simulink model "Model"  (R2015a)
settings: Solver=ode1  StartTime=0.0  StopTime=Inf  FixedStep=0.001  RelTol=1e-3
PostLoadFcn:
  | , if any(exist('dsrtsu_mdlpostloadfcn', 'file') == [2, 3, 6]), try dsrtsu_mdlpostloadfcn('Execute', bdroot); catch fprintf('Error in PostLoadFcn (dsrtsu_mdlpostloadfcn) for model "%s":\n %s\n', bdroot, lasterr); end, end,
libraries: rtilib1104 x9, simulink x6, simulink_extras x3
settings Model: DSRTSU_INTERNAL_RTI_VER=460  DSRTSU_INTERNAL_RTI_TYPE=rti1104  DSRTSU_INTERNAL_RTIFPGA=50  Creator=k19p800a  LastModifiedBy=k19p800a
settings OptimizationCC: BlockReduction=off  OptimizeBlockIOStorage=off  BufferReuse=off  GlobalBufferReuse=off  ExpressionFolding=off  LocalBlockOutputs=off
settings HardwareCC: ProdIntDivRoundTo=Zero  ProdEndianess=BigEndian  ProdHWDeviceType=Generic->Custom  TargetIntDivRoundTo=Zero  TargetEndianess=BigEndian  TargetHWDeviceType=Generic->Custom
settings RTWCC: SystemTargetFile=rti1104.tlc  MakeCommand=make_rti  TemplateMakefile=rti1104.tmf  Description=dSPACE DS1104 Hardware Platform
settings STFCustomTargetCC: GenerateSampleERTMain=off  ParMdlRefBuildCompliant=on  GeneratePreprocessorConditionals=Disable all  ERTCustomFileBanners=off  SupportNonInlinedSFcns=on  SupportVariableSizeSignals=off  MATLABClassNameForMDSCustomization=Simulink.SoftwareTarget.GRTCustomization  GRTInterface=on  SystemTargetFile=rti1104.tlc
settings GRTTargetCC: CompOptLevelCompliant=off  ConcurrentExecutionCompliant=off  CombineOutputUpdateFcns=off  MatFileLogging=off  CPPClassGenCompliant=off  GRTInterface=on  ExtModeMexFile=noextcomm

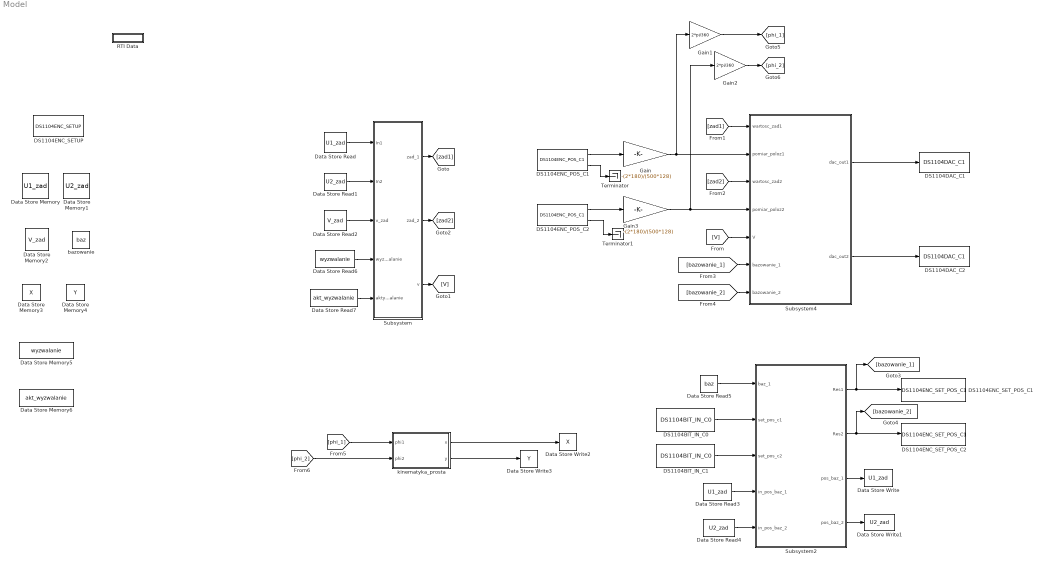
== system Model ==
  DS1104BIT_IN_C0 : rtilib1104/DS1104 MASTER PPC/DS1104BIT_IN_C0  ChannelNo=0  Reserved1=[]  Reserved2=[]  Reserved3=[]  Reserved4=[]  DialogFcn=gui1104bit_in  UnitName={'DS1104BIT_IN_C'}  UnitValues={ 0 }  DSProperties=struct('RTI',struct('Version',uint32(1),'BlockType',struct('isSLSource',uint8(1),'isSLSink',uint8(0),'isHWSource',uint8(1),'isHWSink',uint8(0),'isSetup',uint8(0),'isInline',uint8(1),'isNonInline',uint8(0),'isInterrupt',uint8(0),'isChannelwise',uint8(1)),'IOBoardType','DS1104MASTER','UnitType','BIT','Identifier','BITINCH','DialogType','ML','BlockSet','NONE','SlaveProcessor','NONE'))
  DS1104BIT_IN_C1 : rtilib1104/DS1104 MASTER PPC/DS1104BIT_IN_C0  ChannelNo=1  Reserved1=[]  Reserved2=[]  Reserved3=[]  Reserved4=[]  DialogFcn=gui1104bit_in  UnitName={'DS1104BIT_IN_C'}  UnitValues={ 1 }  DSProperties=struct('RTI',struct('Version',uint32(1),'BlockType',struct('isSLSource',uint8(1),'isSLSink',uint8(0),'isHWSource',uint8(1),'isHWSink',uint8(0),'isSetup',uint8(0),'isInline',uint8(1),'isNonInline',uint8(0),'isInterrupt',uint8(0),'isChannelwise',uint8(1)),'IOBoardType','DS1104MASTER','UnitType','BIT','Identifier','BITINCH','DialogType','ML','BlockSet','NONE','SlaveProcessor','NONE'))
  DS1104DAC_C1 : rtilib1104/DS1104 MASTER PPC/DS1104DAC_C1  ChannelNo=1  InitValue=0  TermMode=0  TermValue=0  Reserved1=[]  Reserved2=[]  Reserved3=[]  Reserved4=[]  DialogFcn=gui1104dac  UnitName={ 'DS1104DAC_C'}  UnitValues={ 1 }  DSProperties=struct('RTI',struct('Version',uint32(1),'BlockType',struct('isSLSource',uint8(0),'isSLSink',uint8(1),'isHWSource',uint8(0),'isHWSink',uint8(1),'isSetup',uint8(0),'isInline',uint8(1),'isNonInline',uint8(0),'isInterrupt',uint8(0),'isChannelwise',uint8(1)),'IOBoardType','DS1104MASTER','UnitType','DAC','Identifier','DAC','DialogType','ML','BlockSet','NONE','SlaveProcessor','NONE'))
  DS1104DAC_C2 : rtilib1104/DS1104 MASTER PPC/DS1104DAC_C1  ChannelNo=2  InitValue=0  TermMode=0  TermValue=0  Reserved1=[]  Reserved2=[]  Reserved3=[]  Reserved4=[]  DialogFcn=gui1104dac  UnitName={ 'DS1104DAC_C'}  UnitValues={2}  DSProperties=struct('RTI',struct('Version',uint32(1),'BlockType',struct('isSLSource',uint8(0),'isSLSink',uint8(1),'isHWSource',uint8(0),'isHWSink',uint8(1),'isSetup',uint8(0),'isInline',uint8(1),'isNonInline',uint8(0),'isInterrupt',uint8(0),'isChannelwise',uint8(1)),'IOBoardType','DS1104MASTER','UnitType','DAC','Identifier','DAC','DialogType','ML','BlockSet','NONE','SlaveProcessor','NONE'))
  DS1104ENC_POS_C1 : rtilib1104/DS1104 MASTER PPC/DS1104ENC_POS_C1  ChannelNo=1  PosValue=0  Reserved1=[]  Reserved2=[]  Reserved3=[]  Reserved4=[]  DialogFcn=gui1104enc_pos  UnitName={'DS1104ENC_POS_C'}  UnitValues={ 1 }  DSProperties=struct('RTI',struct('Version',uint32(1),'BlockType',struct('isSLSource',uint8(1),'isSLSink',uint8(0),'isHWSource',uint8(1),'isHWSink',uint8(0),'isSetup',uint8(0),'isInline',uint8(1),'isNonInline',uint8(0),'isInterrupt',uint8(0),'isChannelwise',uint8(1)),'IOBoardType','DS1104MASTER','UnitType','ENC','Identifier','ENCPOSCH','DialogType','ML','BlockSet','NONE','SlaveProcessor','NONE'))
  DS1104ENC_POS_C2 : rtilib1104/DS1104 MASTER PPC/DS1104ENC_POS_C1  ChannelNo=2  PosValue=0  Reserved1=[]  Reserved2=[]  Reserved3=[]  Reserved4=[]  DialogFcn=gui1104enc_pos  UnitName={'DS1104ENC_POS_C'}  UnitValues={2}  DSProperties=struct('RTI',struct('Version',uint32(1),'BlockType',struct('isSLSource',uint8(1),'isSLSink',uint8(0),'isHWSource',uint8(1),'isHWSink',uint8(0),'isSetup',uint8(0),'isInline',uint8(1),'isNonInline',uint8(0),'isInterrupt',uint8(0),'isChannelwise',uint8(1)),'IOBoardType','DS1104MASTER','UnitType','ENC','Identifier','ENCPOSCH','DialogType','ML','BlockSet','NONE','SlaveProcessor','NONE'))
  DS1104ENC_SETUP : rtilib1104/DS1104 MASTER PPC/DS1104ENC_SETUP  Reserved1=[]  Reserved2=[]  Reserved3=[]  Reserved4=[]  DialogFcn=gui1104enc_setup  UnitName={'DS1104ENC_SETUP'}  UnitValues={ [] }  DSProperties=struct('RTI',struct('Version',uint32(1),'BlockType',struct('isSLSource',uint8(0),'isSLSink',uint8(0),'isHWSource',uint8(0),'isHWSink',uint8(0),'isSetup',uint8(0),'isInline',uint8(1),'isNonInline',uint8(0),'isInterrupt',uint8(0),'isChannelwise',uint8(0)),'IOBoardType','DS1104MASTER','UnitType','ENC','Identifier','ENCSETUP','DialogType','ML','BlockSet','NONE','SlaveProcessor','NONE'))
      settings: SignalType=[0 0]
  DS1104ENC_SET_POS_C1 : rtilib1104/DS1104 MASTER PPC/DS1104ENC_SET_POS_C1  ChannelNo=1  PosValue=0  Reserved1=[]  Reserved2=[]  Reserved3=[]  Reserved4=[]  DialogFcn=gui1104enc_set_pos  UnitName={'DS1104ENC_SET_POS_C'}  UnitValues={ 1 }  DSProperties=struct('RTI',struct('Version',uint32(1),'BlockType',struct('isSLSource',uint8(0),'isSLSink',uint8(1),'isHWSource',uint8(0),'isHWSink',uint8(1),'isSetup',uint8(0),'isInline',uint8(1),'isNonInline',uint8(0),'isInterrupt',uint8(0),'isChannelwise',uint8(1)),'IOBoardType','DS1104MASTER','UnitType','ENC','Identifier','ENCRESET','DialogType','ML','BlockSet','NONE','SlaveProcessor','NONE'))
  DS1104ENC_SET_POS_C2 : rtilib1104/DS1104 MASTER PPC/DS1104ENC_SET_POS_C1  ChannelNo=2  PosValue=0  Reserved1=[]  Reserved2=[]  Reserved3=[]  Reserved4=[]  DialogFcn=gui1104enc_set_pos  UnitName={'DS1104ENC_SET_POS_C'}  UnitValues={2}  DSProperties=struct('RTI',struct('Version',uint32(1),'BlockType',struct('isSLSource',uint8(0),'isSLSink',uint8(1),'isHWSource',uint8(0),'isHWSink',uint8(1),'isSetup',uint8(0),'isInline',uint8(1),'isNonInline',uint8(0),'isInterrupt',uint8(0),'isChannelwise',uint8(1)),'IOBoardType','DS1104MASTER','UnitType','ENC','Identifier','ENCRESET','DialogType','ML','BlockSet','NONE','SlaveProcessor','NONE'))
  Data Store Memory : DataStoreMemory  DataStoreName=U1_zad  ReadBeforeWriteMsg=warning  WriteAfterWriteMsg=warning  WriteAfterReadMsg=warning
  Data Store Memory1 : DataStoreMemory  DataStoreName=U2_zad  ReadBeforeWriteMsg=warning  WriteAfterWriteMsg=warning  WriteAfterReadMsg=warning
  Data Store Memory2 : DataStoreMemory  DataStoreName=V_zad  ReadBeforeWriteMsg=warning  WriteAfterWriteMsg=warning  WriteAfterReadMsg=warning  InitialValue=25
  Data Store Memory3 : DataStoreMemory  DataStoreName=X  ReadBeforeWriteMsg=warning  WriteAfterWriteMsg=warning  WriteAfterReadMsg=warning
  Data Store Memory4 : DataStoreMemory  DataStoreName=Y  ReadBeforeWriteMsg=warning  WriteAfterWriteMsg=warning  WriteAfterReadMsg=warning
  Data Store Memory5 : DataStoreMemory  DataStoreName=wyzwalanie  ReadBeforeWriteMsg=warning  WriteAfterWriteMsg=warning  WriteAfterReadMsg=warning
  Data Store Memory6 : DataStoreMemory  DataStoreName=akt_wyzwalanie  ReadBeforeWriteMsg=warning  WriteAfterWriteMsg=warning  WriteAfterReadMsg=warning
  Data Store Read : DataStoreRead  DataStoreName=U1_zad
  Data Store Read1 : DataStoreRead  DataStoreName=U2_zad
  Data Store Read2 : DataStoreRead  DataStoreName=V_zad
  Data Store Read3 : DataStoreRead  DataStoreName=U1_zad
  Data Store Read4 : DataStoreRead  DataStoreName=U2_zad
  Data Store Read5 : DataStoreRead  DataStoreName=baz
  Data Store Read6 : DataStoreRead  DataStoreName=wyzwalanie
  Data Store Read7 : DataStoreRead  DataStoreName=akt_wyzwalanie
  Data Store Write : DataStoreWrite  DataStoreName=U1_zad
  Data Store Write1 : DataStoreWrite  DataStoreName=U2_zad
  Data Store Write2 : DataStoreWrite  DataStoreName=X
  Data Store Write3 : DataStoreWrite  DataStoreName=Y
  Gain : Gain  Gain=-(2*180)/(500*128)
  Gain1 : Gain  Gain=2*pi/360
  Gain2 : Gain  Gain=2*pi/360
  Gain3 : Gain  Gain=-(2*180)/(500*128)
  RTI Data : Subsystem  Tag=struct('RTIDataServer',struct('RTIDataServerVs','2','RTIModelDescription','struct(''main'',''Model'',''sub'','''',''isMp'',0)'))  LoadFcn="if exist('rtidc'), try,  rtidc('DataHostBlockClbLoad', gcbh); catch, disp(['Warning: ''LoadFcn'' for RTI Data block failed: ' lasterr]); end, end,"  mask(RTI_DATA_HOST){}
      mask help:
      | RTI Data Block.
      | This block is used by RTI to store internal model-dependent data.
      | Please keep this block on the root level of the model. Deleting this block will result in data loss.
      |
      | NEVER DELETE OR COPY THIS BLOCK!
      settings: CopyFcn="if exist('rtidc'), try,  rtidc('DataHostBlockClbCopy', gcbh); catch, disp(['Warning: ''CopyFcn'' for RTI Data block failed: ' lasterr]); end, end,"  DeleteFcn="if exist('rtidc'), try,  rtidc('DataHostBlockClbDelete', gcbh); catch, disp(['Warning: ''DeleteFcn'' for RTI Data block failed: ' lasterr]); end, end,"  ModelCloseFcn="if exist('rtidc'), try,  rtidc('DataHostBlockClbModelClose', gcbh); catch, disp(['Warning: ''ModelCloseFcn'' for RTI Data block failed: ' lasterr]); end, end,"  PreSaveFcn="if exist('rtidc'), try,  rtidc('DataHostBlockClbPreSave', gcbh); catch, disp(['Warning: ''PreSaveFcn'' for RTI Data block failed: ' lasterr]); end, end,"  PostSaveFcn="if exist('rtidc'), try,  rtidc('DataHostBlockClbPostSave', gcbh); catch, disp(['Warning: ''PostSaveFcn'' for RTI Data block failed: ' lasterr]); end, end,"  NameChangeFcn="if exist('rtidc'), try,  rtidc('DataHostBlockClbNameChange', gcbh); catch, disp(['Warning: ''NameChangeFcn'' for RTI Data block failed: ' lasterr]); end, end,"
      mask Help:
      | RTI Data Block.
      | This block is used by RTI to store internal model-dependent data.
      | Please keep this block on the root level of the model. Deleting this block will result in data loss.
      | 
      | NEVER DELETE OR COPY THIS BLOCK!
      mask Display:
      | text(0.5, 0.5, 'RTI Data', 'HorizontalAlignment', 'center');
      | plot([1 0]);
  Subsystem : Subsystem
  Subsystem2 : Subsystem
  Subsystem4 : Subsystem
  Terminator : Terminator
  Terminator1 : Terminator
  bazowanie : DataStoreMemory  DataStoreName=baz  ReadBeforeWriteMsg=warning  WriteAfterWriteMsg=warning  WriteAfterReadMsg=warning
  kinematyka_prosta : Subsystem
  wires:
  DS1104ENC_POS_C1/2 -> Terminator/1
  DS1104ENC_POS_C1/1 -> Gain/1
  Data Store Read/1 -> Subsystem/1(In1)
  Data Store Read1/1 -> Subsystem/2(In2)
  Data Store Read2/1 -> Subsystem/3(v_zad)
  Subsystem/1(zad_1) -> [zad1]
  DS1104ENC_POS_C2/1 -> Gain3/1
  DS1104ENC_POS_C2/2 -> Terminator1/1
  Gain/1 -> Gain1/1, Subsystem4/2(pomiar_poloz1)
  Gain3/1 -> Gain2/1, Subsystem4/4(pomiar_poloz2)
  Subsystem/3(v) -> [V]
  [V] -> Subsystem4/5(V)
  [zad1] -> Subsystem4/1(wartosc_zad1)
  Subsystem/2(zad_2) -> [zad2]
  [zad2] -> Subsystem4/3(wartosc_zad2)
  Subsystem2/3(pos_baz_1) -> Data Store Write/1
  Subsystem2/4(pos_baz_2) -> Data Store Write1/1
  Data Store Read3/1 -> Subsystem2/4(in_pos_baz_1)
  Data Store Read4/1 -> Subsystem2/5(in_pos_baz_2)
  Data Store Read5/1 -> Subsystem2/1(baz_1)
  Subsystem2/1(Res1) -> DS1104ENC_SET_POS_C1/Trigger, [bazowanie_1]
  Subsystem2/2(Res2) -> DS1104ENC_SET_POS_C2/Trigger, [bazowanie_2]
  [bazowanie_1] -> Subsystem4/6(bazowanie_1)
  [bazowanie_2] -> Subsystem4/7(bazowanie_2)
  Gain1/1 -> [phi_1]
  Gain2/1 -> [phi_2]
  [phi_1] -> kinematyka_prosta/1(phi1)
  [phi_2] -> kinematyka_prosta/2(phi2)
  kinematyka_prosta/1(x) -> Data Store Write2/1
  kinematyka_prosta/2(y) -> Data Store Write3/1
  Data Store Read6/1 -> Subsystem/4("wyzwalanie ")
  Data Store Read7/1 -> Subsystem/5(aktywuj_wyzwalanie)
  DS1104BIT_IN_C0/1 -> Subsystem2/2(set_pos_c1)
  DS1104BIT_IN_C1/1 -> Subsystem2/3(set_pos_c2)
  Subsystem4/2(dac_out2) -> DS1104DAC_C2/1
  Subsystem4/1(dac_out1) -> DS1104DAC_C1/1

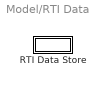
== system Model/RTI Data ==
  RTI Data Store : Subsystem  Tag="struct('private',struct('version',struct('dsVer',uint32(2),'dsVerCreation',uint32(2),'RTI',struct('ver','7.4','type','RTI1104')),'access',struct('type','Model','isPerm',1,'created',['08-Apr-2019 09:21:49'],'modified',['15-Apr-2019 09:27:02'],'location','')),'public',struct('main',struct('data',[]),'sub',struct('name',{{'Model'}},'data',{{struct('TH',struct('thTaskInfo',struct('taskType',{'TIMER','HWINT','TMRINT','SWINT','GLINT'},'tasksNumOf',{1,0,0,0,0},'srcIds',{{'TIMERA'},{},{},{},{}},'taskNames',{{['Timer Task 1']},{},{},{},{}})),'th_tc',struct('dataType','TASK','taskGroupId','','taskGroupList',{{}},'taskSchedulingPolicy','FCFS','taskType','TIMER','blkh',-1,'srcId','TIMERA','srcSgnName',['Timer A interrupt'],'srcCpuName','','taskName',['Timer Task 1  [0.001] s'],'taskNameDisplayExt','','smplTime',0.001,'smplTimeOffs',0,'hasFixedPriority',0,'priority',1,'hasFixedOvc',0,'ovcType',1,'ovcMax',1),'tc_th',struct('dataType','TASK','taskGroupId','','taskGroupList',{{}},'taskSchedulingPolicy','FCFS','taskType','TIMER','blkh',-1,'srcId','TIMERA','srcSgnName',['Timer A interrupt'],'srcCpuName','','taskName',['Timer Task 1  [0.001] s'],'taskNameDisplayExt','','smplTime',0.001,'smplTimeOffs',0,'hasFixedPriority',0,'priority',1,'hasFixedOvc',0,'ovcType',1,'ovcMax',1))}})))"  mask(RTI_DATA_STORE){}
      mask help:
      | RTI Data Store Block. This block is used by RTI to store internal model dependent data. Deleting this block will result in data loss.
      |
      | NEVER DELETE, COPY, OR MODIFY THIS BLOCK!
      mask Help:
      | RTI Data Store Block. This block is used by RTI to store internal model dependent data. Deleting this block will result in data loss.
      | 
      | NEVER DELETE, COPY, OR MODIFY THIS BLOCK!
      mask Display: text(0.5, 0.5, ' ', 'HorizontalAlignment', 'center');

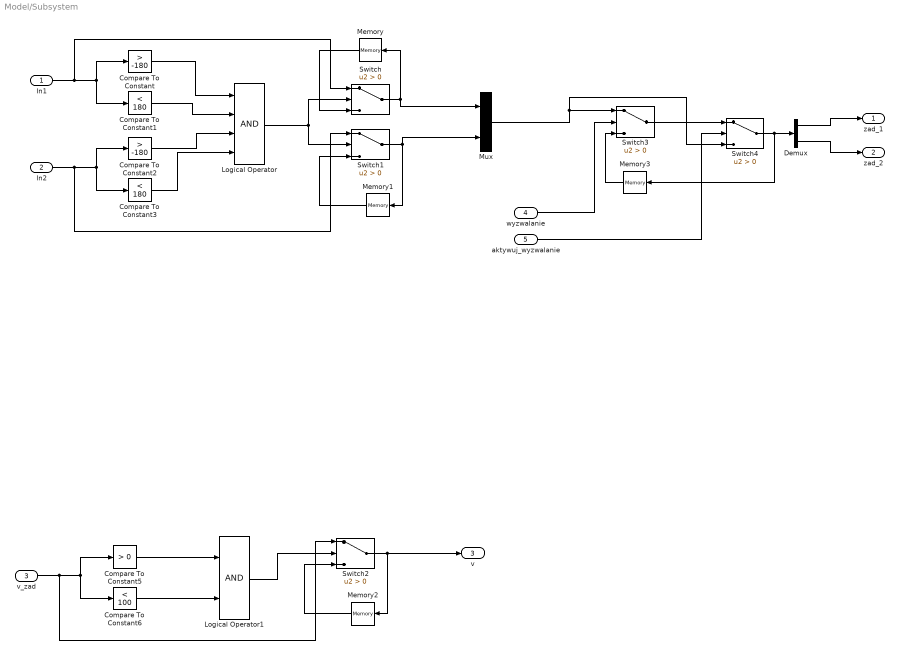
== system Model/Subsystem ==
  In1 : Inport
  In2 : Inport  Port=2
  v_zad : Inport  Port=3
  "wyzwalanie " : Inport  Port=4
  aktywuj_wyzwalanie : Inport  Port=5
  Compare To Constant : simulink/Logic and Bit Operations/Compare To Constant  relop=>  const=-180  OutDataTypeStr=boolean
  Compare To Constant1 : simulink/Logic and Bit Operations/Compare To Constant  relop=<  const=180  OutDataTypeStr=boolean
  Compare To Constant2 : simulink/Logic and Bit Operations/Compare To Constant  relop=>  const=-180  OutDataTypeStr=boolean
  Compare To Constant3 : simulink/Logic and Bit Operations/Compare To Constant  relop=<  const=180  OutDataTypeStr=boolean
  Compare To Constant5 : simulink/Logic and Bit Operations/Compare To Constant  relop=>  const=0  OutDataTypeStr=boolean
  Compare To Constant6 : simulink/Logic and Bit Operations/Compare To Constant  relop=<  const=100  OutDataTypeStr=boolean
  Demux : Demux  Outputs=2
  Logical Operator : Logic  Inputs=4  AllPortsSameDT=off
  Logical Operator1 : Logic  AllPortsSameDT=off
  Memory{,1..3} (4 alike) : Memory
  Mux : Mux  Inputs=2
  Switch{,1..4} (5 alike) : Switch  Criteria=u2 > Threshold
  zad_1 : Outport
  zad_2 : Outport  Port=2
  v : Outport  Port=3
  wires:
  Memory1/1 -> Switch1/3
  Compare To Constant2/1 -> Logical Operator/3
  Memory/1 -> Switch/3
  Compare To Constant1/1 -> Logical Operator/2
  Switch1/1 -> Mux/2, Memory1/1
  Switch/1 -> Memory/1, Mux/1
  Logical Operator/1 -> Switch1/2, Switch/2
  In1/1 -> Switch/1, Compare To Constant/1, Compare To Constant1/1
  In2/1 -> Switch1/1, Compare To Constant3/1, Compare To Constant2/1
  Compare To Constant/1 -> Logical Operator/1
  Compare To Constant3/1 -> Logical Operator/4
  Memory2/1 -> Switch2/3
  Compare To Constant5/1 -> Logical Operator1/1
  Switch2/1 -> Memory2/1, v/1
  Logical Operator1/1 -> Switch2/2
  v_zad/1 -> Compare To Constant5/1, Compare To Constant6/1, Switch2/1
  Compare To Constant6/1 -> Logical Operator1/2
  Mux/1 -> Switch4/3, Switch3/1
  Switch3/1 -> Switch4/1
  Memory3/1 -> Switch3/3
  "wyzwalanie "/1 -> Switch3/2
  aktywuj_wyzwalanie/1 -> Switch4/2
  Switch4/1 -> Memory3/1, Demux/1
  Demux/1 -> zad_1/1
  Demux/2 -> zad_2/1

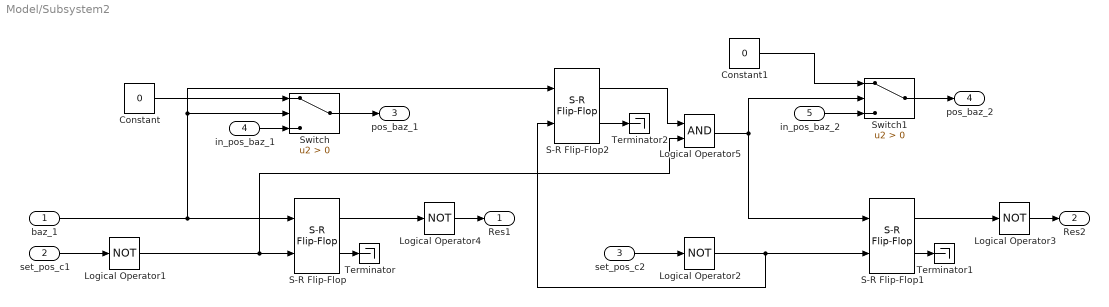
== system Model/Subsystem2 ==
  baz_1 : Inport
  set_pos_c1 : Inport  Port=2
  set_pos_c2 : Inport  Port=3
  in_pos_baz_1 : Inport  Port=4
  in_pos_baz_2 : Inport  Port=5
  Constant : Constant  Value=0
  Constant1 : Constant  Value=0
  Logical Operator{1..4} (4 alike) : Logic  Operator=NOT  AllPortsSameDT=off
  Logical Operator5 : Logic  AllPortsSameDT=off
  S-R Flip-Flop : simulink_extras/Flip Flops/S-R Flip-Flop  initial_condition=0
  S-R Flip-Flop1 : simulink_extras/Flip Flops/S-R Flip-Flop  initial_condition=0
  S-R Flip-Flop2 : simulink_extras/Flip Flops/S-R Flip-Flop  initial_condition=0
  Switch : Switch  Criteria=u2 > Threshold
  Switch1 : Switch  Criteria=u2 > Threshold
  Terminator : Terminator
  Terminator1 : Terminator
  Terminator2 : Terminator
  Res1 : Outport
  Res2 : Outport  Port=2
  pos_baz_1 : Outport  Port=3
  pos_baz_2 : Outport  Port=4
  wires:
  S-R Flip-Flop1/1 -> Logical Operator3/1
  baz_1/1 -> S-R Flip-Flop/1, S-R Flip-Flop2/1, Switch/2
  S-R Flip-Flop/1 -> Logical Operator4/1
  S-R Flip-Flop/2 -> Terminator/1
  S-R Flip-Flop1/2 -> Terminator1/1
  Logical Operator4/1 -> Res1/1
  Logical Operator3/1 -> Res2/1
  Constant/1 -> Switch/1
  Switch/1 -> pos_baz_1/1
  Switch1/1 -> pos_baz_2/1
  set_pos_c2/1 -> Logical Operator2/1
  in_pos_baz_2/1 -> Switch1/3
  in_pos_baz_1/1 -> Switch/3
  set_pos_c1/1 -> Logical Operator1/1
  Logical Operator1/1 -> Logical Operator5/2, S-R Flip-Flop/2
  Logical Operator2/1 -> S-R Flip-Flop2/2, S-R Flip-Flop1/2
  Constant1/1 -> Switch1/1
  S-R Flip-Flop2/1 -> Logical Operator5/1
  Logical Operator5/1 -> S-R Flip-Flop1/1, Switch1/2
  S-R Flip-Flop2/2 -> Terminator2/1

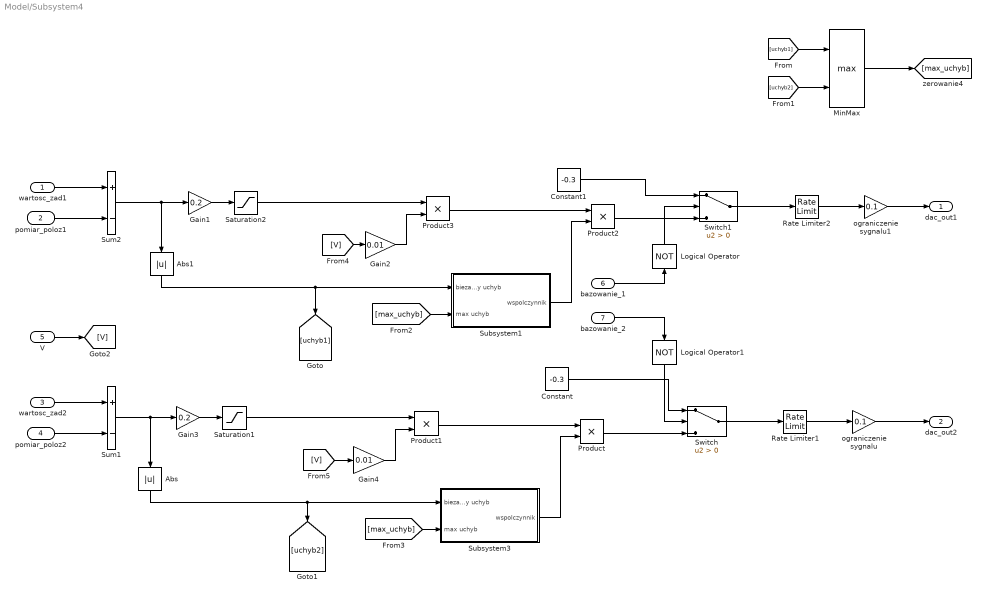
== system Model/Subsystem4 ==
  wartosc_zad1 : Inport
  pomiar_poloz1 : Inport  Port=2
  wartosc_zad2 : Inport  Port=3
  pomiar_poloz2 : Inport  Port=4
  V : Inport  Port=5
  bazowanie_1 : Inport  Port=6
  bazowanie_2 : Inport  Port=7
  Abs : Abs
  Abs1 : Abs
  Constant : Constant  Value=-0.3
  Constant1 : Constant  Value=-0.3
  Gain1 : Gain  Gain=0.2
  Gain2 : Gain  Gain=0.01
  Gain3 : Gain  Gain=0.2
  Gain4 : Gain  Gain=0.01
  Logical Operator : Logic  Operator=NOT  AllPortsSameDT=off
  Logical Operator1 : Logic  Operator=NOT  AllPortsSameDT=off
  MinMax : MinMax  Function=max  Inputs=2
  Product{,1..3} (4 alike) : Product
  Rate Limiter1 : RateLimiter  RisingSlewLimit=50  FallingSlewLimit=-50  SampleTimeMode=inherited
  Rate Limiter2 : RateLimiter  RisingSlewLimit=50  FallingSlewLimit=-50  SampleTimeMode=inherited
  Saturation1 : Saturate  UpperLimit=3  LowerLimit=-3
  Saturation2 : Saturate  UpperLimit=3  LowerLimit=-3
  Subsystem1 : Subsystem
  Subsystem3 : Subsystem
  Sum1 : Sum  Inputs=+-
  Sum2 : Sum  Inputs=+-
  Switch : Switch  Criteria=u2 > Threshold
  Switch1 : Switch  Criteria=u2 > Threshold
  ograniczenie sygnalu : Gain  Gain=0.1
  ograniczenie sygnalu1 : Gain  Gain=0.1
  dac_out1 : Outport
  dac_out2 : Outport  Port=2
  wires:
  pomiar_poloz2/1 -> Sum1/2
  wartosc_zad2/1 -> Sum1/1
  Gain3/1 -> Saturation1/1
  Sum1/1 -> Abs/1, Gain3/1
  Rate Limiter1/1 -> ograniczenie sygnalu/1
  ograniczenie sygnalu/1 -> dac_out2/1
  Constant/1 -> Switch/1
  Switch/1 -> Rate Limiter1/1
  Abs/1 -> Subsystem3/1(biezacy uchyb), [uchyb2]
  [max_uchyb] -> Subsystem3/2(max uchyb)
  Product/1 -> Switch/3
  Subsystem3/1(wspolczynnik) -> Product/2
  Saturation1/1 -> Product1/1
  Product1/1 -> Product/1
  [V] -> Gain4/1
  Gain4/1 -> Product1/2
  pomiar_poloz1/1 -> Sum2/2
  wartosc_zad1/1 -> Sum2/1
  Gain1/1 -> Saturation2/1
  Sum2/1 -> Gain1/1, Abs1/1
  Rate Limiter2/1 -> ograniczenie sygnalu1/1
  ograniczenie sygnalu1/1 -> dac_out1/1
  Constant1/1 -> Switch1/1
  Switch1/1 -> Rate Limiter2/1
  Abs1/1 -> Subsystem1/1(biezacy uchyb), [uchyb1]
  [max_uchyb] -> Subsystem1/2(max uchyb)
  Product2/1 -> Switch1/3
  Subsystem1/1(wspolczynnik) -> Product2/2
  Saturation2/1 -> Product3/1
  Product3/1 -> Product2/1
  [V] -> Gain2/1
  Gain2/1 -> Product3/2
  MinMax/1 -> [max_uchyb]
  [uchyb1] -> MinMax/1
  [uchyb2] -> MinMax/2
  V/1 -> [V]
  Logical Operator/1 -> Switch1/2
  Logical Operator1/1 -> Switch/2
  bazowanie_2/1 -> Logical Operator1/1
  bazowanie_1/1 -> Logical Operator/1

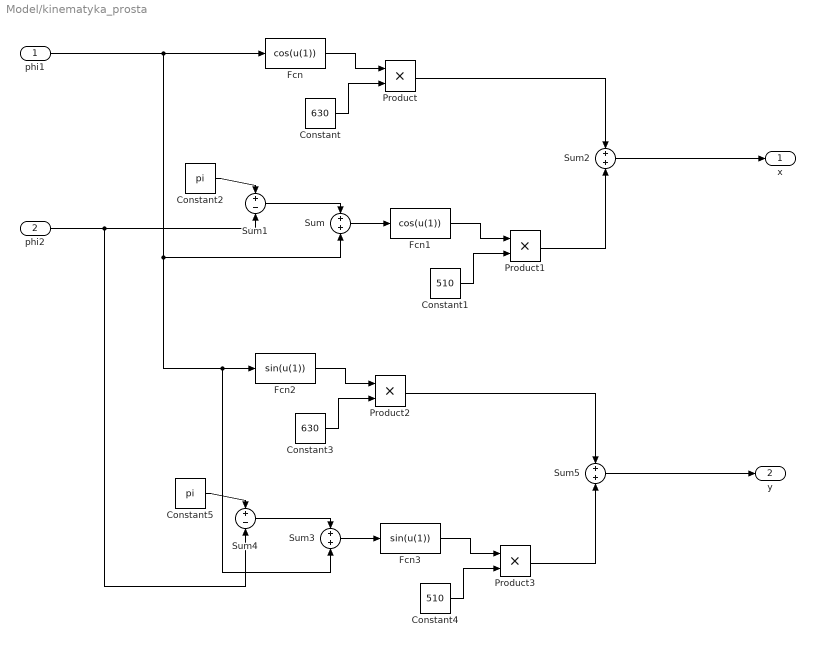
== system Model/kinematyka_prosta ==
  phi1 : Inport
  phi2 : Inport  Port=2
  Constant : Constant  Value=630
  Constant1 : Constant  Value=510
  Constant2 : Constant  Value=pi
  Constant3 : Constant  Value=630
  Constant4 : Constant  Value=510
  Constant5 : Constant  Value=pi
  Fcn : Fcn  Expr=cos(u(1))
  Fcn1 : Fcn  Expr=cos(u(1))
  Fcn2 : Fcn  Expr=sin(u(1))
  Fcn3 : Fcn  Expr=sin(u(1))
  Product{,1..3} (4 alike) : Product
  Sum{,2..3,5} (4 alike) : Sum
  Sum1 : Sum  Inputs=+-
  Sum4 : Sum  Inputs=+-
  x : Outport
  y : Outport  Port=2
  wires:
  Fcn/1 -> Product/1
  Constant2/1 -> Sum1/1
  Constant3/1 -> Product2/2
  Fcn2/1 -> Product2/1
  Product2/1 -> Sum5/1
  Fcn3/1 -> Product3/1
  Sum1/1 -> Sum/1
  Fcn1/1 -> Product1/1
  Constant5/1 -> Sum4/1
  Product3/1 -> Sum5/2
  Constant4/1 -> Product3/2
  phi1/1 -> Sum3/2, Fcn2/1, Sum/2, Fcn/1
  Sum3/1 -> Fcn3/1
  Sum4/1 -> Sum3/1
  phi2/1 -> Sum4/2, Sum1/2
  Constant1/1 -> Product1/2
  Sum/1 -> Fcn1/1
  Constant/1 -> Product/2
  Product1/1 -> Sum2/2
  Sum2/1 -> x/1
  Product/1 -> Sum2/1
  Sum5/1 -> y/1

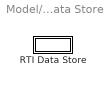
== system Model/RTI Data/RTI Data Store ==
  RTI Data Store : Subsystem  mask(RTI_DATA_STORE){}
      mask help:
      | RTI Data Store Block. This block is used by RTI to store internal model dependent data. Deleting this block will result in data loss.
      |
      | NEVER DELETE, COPY, OR MODIFY THIS BLOCK!
      mask Help:
      | RTI Data Store Block. This block is used by RTI to store internal model dependent data. Deleting this block will result in data loss.
      | 
      | NEVER DELETE, COPY, OR MODIFY THIS BLOCK!
      mask Display: text(0.5, 0.5, ' ', 'HorizontalAlignment', 'center');

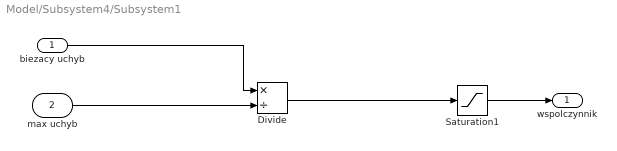
== system Model/Subsystem4/Subsystem1 ==
  biezacy uchyb : Inport
  max uchyb : Inport  Port=2
  Divide : Product  Inputs=*/
  Saturation1 : Saturate  UpperLimit=1  LowerLimit=0.05
  wspolczynnik : Outport
  wires:
  Saturation1/1 -> wspolczynnik/1
  Divide/1 -> Saturation1/1
  biezacy uchyb/1 -> Divide/1
  max uchyb/1 -> Divide/2

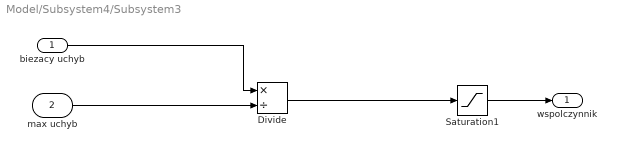
== system Model/Subsystem4/Subsystem3 ==
  biezacy uchyb : Inport
  max uchyb : Inport  Port=2
  Divide : Product  Inputs=*/
  Saturation1 : Saturate  UpperLimit=1  LowerLimit=0.05
  wspolczynnik : Outport
  wires:
  max uchyb/1 -> Divide/2
  biezacy uchyb/1 -> Divide/1
  Divide/1 -> Saturation1/1
  Saturation1/1 -> wspolczynnik/1

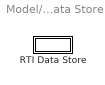
== system Model/RTI Data/RTI Data Store/RTI Data Store ==
  RTI Data Store : Subsystem  mask(RTI_DATA_STORE){}
      mask help:
      | RTI Data Store Block. This block is used by RTI to store internal model dependent data. Deleting this block will result in data loss.
      |
      | NEVER DELETE, COPY, OR MODIFY THIS BLOCK!
      mask Help:
      | RTI Data Store Block. This block is used by RTI to store internal model dependent data. Deleting this block will result in data loss.
      | 
      | NEVER DELETE, COPY, OR MODIFY THIS BLOCK!
      mask Display: text(0.5, 0.5, ' ', 'HorizontalAlignment', 'center');

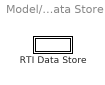
== system Model/RTI Data/RTI Data Store/RTI Data Store/RTI Data Store ==
  RTI Data Store : Subsystem  mask(RTI_DATA_STORE){}
      mask help:
      | RTI Data Store Block. This block is used by RTI to store internal model dependent data. Deleting this block will result in data loss.
      |
      | NEVER DELETE, COPY, OR MODIFY THIS BLOCK!
      mask Help:
      | RTI Data Store Block. This block is used by RTI to store internal model dependent data. Deleting this block will result in data loss.
      | 
      | NEVER DELETE, COPY, OR MODIFY THIS BLOCK!
      mask Display: text(0.5, 0.5, ' ', 'HorizontalAlignment', 'center');

== system Model/RTI Data/RTI Data Store/RTI Data Store/RTI Data Store/RTI Data Store ==
